simulink model "sl_subsys_swerr1"  (Simulink 6.0)
settings: Solver=FixedStepDiscrete  StartTime=0.0  StopTime=10.0  FixedStep=1  RelTol=1e-3
settings Model: CovMetricSettings=d  Creator=The MathWorks Inc.  LastModifiedBy=batserve  ExtModeAutoUpdateStatusClock=off
settings OptimizationCC: BlockReduction=off  BooleanDataType=off
settings DebuggingCC: CheckExecutionContextPreStartOutputMsg=on  CheckExecutionContextRuntimeOutputMsg=on  SolverPrmCheckMsg=none
settings HardwareCC: TargetUnknown=on

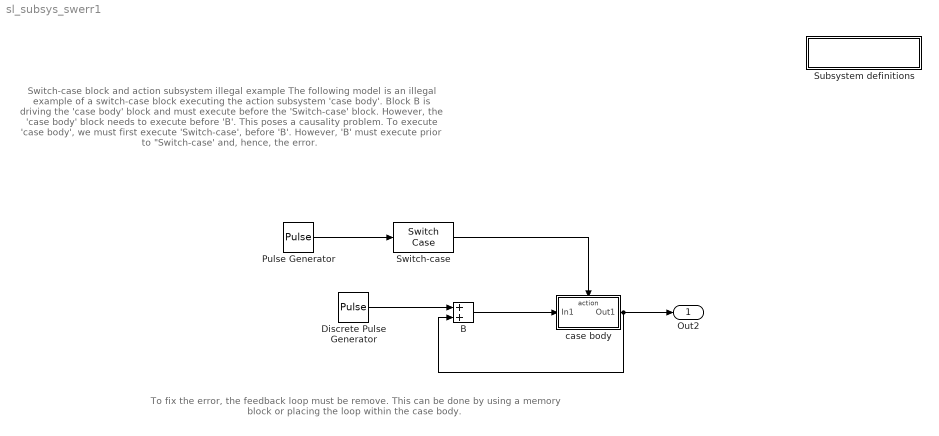
== system sl_subsys_swerr1 ==
  note: To fix the error, the feedback loop must be remove. This can be done by
      | using a memory block or placing the loop within the case body.
  note: Switch-case block and action subsystem illegal example
      |
      | The following model is an illegal example of a switch-case block executing
      | the action subsystem 'case body'. Block B is driving the 'case body' block and
      | must execute before the 'Switch-case' block. However, the 'case body' block needs to execute
      | before 'B'. This poses a causality problem.  To execute 'case body', we must
      | first execute 'Switch-case', before 'B'. However, 'B' must execute prior to
      | "Switch-case' and, hence, the error.
  " Subsystem definitions" : Subsystem  PropExecContextAcrossSSBoundary=on
      settings: OpenFcn=helpview([matlabroot,'/toolbox/simulink/simdemos/sl_subsys_definitions.html']);
      mask Display: disp('Subsystem\ndefinitions')
  B : Sum  SaturateOnIntegerOverflow=on  InputSameDT=on
  Discrete Pulse Generator : DiscretePulseGenerator
  Pulse Generator : DiscretePulseGenerator
  Switch-case : SwitchCase  CaseShowDefault=off
  case body : Subsystem  TreatAsAtomicUnit=on  PropExecContextAcrossSSBoundary=on
  Out2 : Outport
  wires:
  Switch-case/1 -> case body/Action
  B/1 -> case body/1(In1)
  Pulse Generator/1 -> Switch-case/1
  Discrete Pulse Generator/1 -> B/1
  case body/1(Out1) -> B/2, Out2/1

== system sl_subsys_swerr1/ Subsystem definitions ==

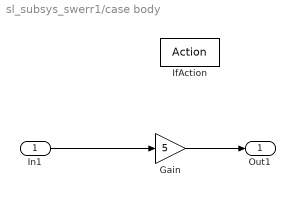
== system sl_subsys_swerr1/case body ==
  In1 : Inport  Port=1  LatchInput=off
  IfAction : ActionPort  ActionType=case
  Gain : Gain  Gain=5  SaturateOnIntegerOverflow=on
  Out1 : Outport
  wires:
  In1/1 -> Gain/1
  Gain/1 -> Out1/1
